simulink model "untitled"  (Simulink 7.6)
settings: Solver=ode3  StartTime=0.0  StopTime=10.0  FixedStep=0.0001  RelTol=1e-3
libraries: simulink x1
settings Model: Creator=student  LastModifiedBy=student

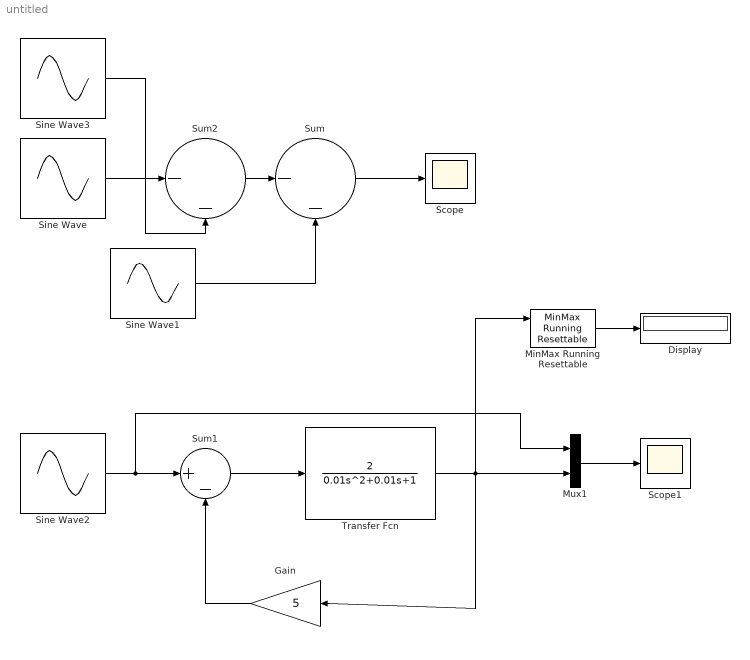
== system untitled ==
  Display : Display
  Gain : Gain  Gain=5
  MinMax Running Resettable : simulink/Math Operations/MinMax Running Resettable  SystemSampleTime=-1  Function=max  vinit=0.0
  Mux1 : Mux  Inputs=2
  Scope : Scope
      settings: MaxDataPoints=500000
  Scope1 : Scope
      settings: MaxDataPoints=10000000
  Sine Wave : Sin  Amplitude=2  SampleTime=0
  Sine Wave1 : Sin  Amplitude=3  Frequency=5  SampleTime=0
  Sine Wave2 : Sin  Amplitude=2.7  Frequency=16  SampleTime=0
  Sine Wave3 : Sin  Amplitude=2  Frequency=9  SampleTime=0
  Sum : Sum  Inputs=|--
  Sum1 : Sum  Inputs=|+-
  Sum2 : Sum  Inputs=|--
  Transfer Fcn : TransferFcn  Numerator=[2]  Denominator=[0.01 0.01 1]
  wires:
  Sine Wave1/1 -> Sum/2
  Sum/1 -> Scope/1
  Gain/1 -> Sum1/2
  Sum1/1 -> Transfer Fcn/1
  Mux1/1 -> Scope1/1
  Sine Wave2/1 -> Sum1/1, Mux1/1
  Transfer Fcn/1 -> Mux1/2, Gain/1, MinMax Running Resettable/1
  MinMax Running Resettable/1 -> Display/1
  Sum2/1 -> Sum/1
  Sine Wave/1 -> Sum2/1
  Sine Wave3/1 -> Sum2/2
